simulink model "PubIfDecisionLM_MDL"  (R2020b)
settings: configuration reference "DspaceConfig" (kept outside this file)
PostLoadFcn:
  | if any(exist('dsrtsu_mdlpostloadfcn', 'file') ~= 0), dsrtsu_mdlpostloadfcn('Execute', bdroot); end
InitFcn:
  | , if any(exist('dsmpb_private', 'file') ~= 0), dsmpb_private('dsmpb_mdlclblib', 'Init', bdroot); end,
undefined symbols (not defined in the file or in its folder): OFM_OBJ_FUSIONTYPE_E, OFM_OBJ_MOVINGSTATE_E, OFM_OBJ_ORIENTATION_E, OFM_OBJ_TYPE_E, P_LM_Cyc, P_LM_EMLHistKapRcdBufSize, P_LM_EMLHistTrajBaseDis, P_LM_EMLHistTrajPNum, P_LM_EMLKapCorrMaxThre, P_LM_EMLMinKapThre, P_LM_EMLPathDisDiffThre, P_LM_EMLQuaFiltPar, P_LM_EMLTurnActKapThre, P_LM_EMLValidQuaThre, P_LM_FntPath1Disgap, P_LM_FntPath1MinDis, P_LM_FntPath1Timegap, P_LM_FntPath2Disgap, P_LM_FntPath2MinDis, P_LM_FntPath2Timegap, P_LM_FntPath3Disgap, P_LM_FntPath3MinDis, P_LM_FntPath3Timegap, P_LM_FusBLParFiltP, P_LM_FusEVDifC2Thre, P_LM_FusEVOPath1AllVSLDisThre, P_LM_FusEVOPath1AllVSLLostNumThre, P_LM_FusEVOPath1AllVSLQuaThre, P_LM_FusEVOPath1OTLFacNLC, P_LM_FusOTLQuaThre, P_LM_FusOTLSW, P_LM_FusParC0Index, P_LM_FusParC1Index, P_LM_FusParC2Index, P_LM_FusParC3Index, P_LM_FusVSLQuaThre, P_LM_FusVSLSW, P_LM_FusVSLValidSteerWheerAngThre, P_LM_FusVSLValidVxvThre, P_LM_LaneWidth, P_LM_OTLBufTPInfoEvaFactor, P_LM_OTLObjNum, P_LM_OTLObjSelectAgeThre, P_LM_OTLObjSelectDxAssessVx, P_LM_OTLObjSelectDxThre, P_LM_OTLObjSelectVxThre, P_LM_OTLObjSelectVyAssessDx, P_LM_OTLObjSelectVyThre, P_LM_OTLTrajPntBaseDis, P_LM_OTLTrajStdThre, P_LM_VSLAvailLineNum, P_LM_VSLBLSDiffThre, P_LM_VSLBLSDisRatio, P_LM_VSLFusBLParFiltP_C1, P_LM_VSLFusBLParFiltP_C2, P_LM_VSLFusBLParFiltP_C3, P_LM_VSLFusBLParFiltP_Quality, P_LM_VSLHistTrajBaseDis, P_LM_VSLHistTrajPNum, P_LM_VSLLCC0diff ... (+18)
libraries: simulink x145, LM_LIB x43
(part 22 of 24)

== matlab function PubIfDecisionLM_MDL/Subsystem2/LM_OTL/LM_OTL_MovObjTrajFit/LM_OTL_BufTPAssess/LM_OTL_BufTrajEva/Subsystem7/MATLAB Function1 ==
  data: Offset output; Flg output; LM_OTLBufValidInfo input; LM_OTLDxVect input; LM_OTLDyVect input; LM_OTLSPPos input; LM_OTLEPPos input; LM_FntPath1Dis input; LM_FntPath2Dis input; LM_FntPath3Dis input; TpValidNum output; SPValidPos output; P_LM_OTLTrajStdThre input
function [Offset,Flg,TpValidNum,SPValidPos] = fcn(LM_OTLBufValidInfo,LM_OTLDxVect,LM_OTLDyVect,LM_OTLSPPos,LM_OTLEPPos,LM_FntPath1Dis,LM_FntPath2Dis,LM_FntPath3Dis, P_LM_OTLTrajStdThre)


%%第一段前车道线取点
Offset=single(zeros(3,1));
Flg=uint8(zeros(3,1));
TpValidNum=uint8(zeros(3,1));
SPValidPos=uint8(zeros(3,1));
t_pnum=uint8(0);
t_sumy=single(0);
t_sumerry=single(0);
t_index=uint8(0);
if LM_OTLBufValidInfo(1)~=0
    if LM_OTLEPPos>=LM_OTLSPPos
        for i=LM_OTLSPPos:LM_OTLEPPos
            if LM_OTLDxVect(i)>0&&LM_OTLDxVect(i)<=LM_FntPath1Dis
                t_pnum=t_pnum+uint8(1);
                t_index=i;
                t_sumy=t_sumy+LM_OTLDyVect(i);
            end
        end
        t_mean=t_sumy/single(t_pnum);
        SPValidPos(1)=t_index-t_pnum+uint8(1);
        for i=t_index:-1:SPValidPos(1)
            t_error=(LM_OTLDyVect(i)-t_mean)^2;
            t_sumerry=t_sumerry+t_error;
        end
        if sqrt(t_sumerry/single(t_pnum))<=P_LM_OTLTrajStdThre
           Offset(1)=t_mean;
           Flg(1)=uint8(1);
           TpValidNum(1)=t_pnum;
        end
    elseif LM_OTLEPPos<LM_OTLSPPos
        for i=LM_OTLSPPos:80
            if LM_OTLDxVect(i)>0&&LM_OTLDxVect(i)<=LM_FntPath1Dis
                t_pnum=t_pnum+uint8(1);
                t_index=i;
                t_sumy=t_sumy+LM_OTLDyVect(i);
            end
        end
        for i=1:LM_OTLEPPos 
            if LM_OTLDxVect(i)>0&&LM_OTLDxVect(i)<=LM_FntPath1Dis
                t_pnum=t_pnum+uint8(1);
                t_index=i;
                t_sumy=t_sumy+LM_OTLDyVect(i);
            end
        end
        SPValidPos(1)=uint8(81)+t_index-t_pnum;
        t_mean=t_sumy/single(t_pnum);
        if SPValidPos(1)>80
            SPValidPos(1)=SPValidPos(1)-80;
        end
        if (SPValidPos(1)>=LM_OTLSPPos&&t_index>=LM_OTLSPPos)||(SPValidPos(1)<LM_OTLSPPos&&t_index<LM_OTLSPPos)
            for i=t_index:-1:SPValidPos(1)
                t_error=(LM_OTLDyVect(i)-t_mean)^2;
                t_sumerry=t_sumerry+t_error;
            end
        else
            for i=1:t_index
                t_error=(LM_OTLDyVect(i)-t_mean)^2;
                t_sumerry=t_sumerry+t_error;
            end
            for i=80:-1:SPValidPos(1)
                 t_error=(LM_OTLDyVect(i)-t_mean)^2;
                t_sumerry=t_sumerry+t_error;
            end
        end
        if sqrt(t_sumerry/single(t_pnum))<=P_LM_OTLTrajStdThre
           Offset(1)=t_mean;
           Flg(1)=uint8(1);
           TpValidNum(1)=t_pnum;
        end           
    end
end
%%第二段前车道线取点
t_pnum=uint8(0);
t_sumy=single(0);
t_sumerry=single(0);
t_index=uint8(0);
if LM_OTLBufValidInfo(2)~=0
    if LM_OTLEPPos>=LM_OTLSPPos
        for i=LM_OTLSPPos:LM_OTLEPPos
            if LM_OTLDxVect(i)>LM_FntPath1Dis&&LM_OTLDxVect(i)<=LM_FntPath2Dis
                t_pnum=t_pnum+uint8(1);
                t_index=i;
                t_sumy=t_sumy+LM_OTLDyVect(i);
            end
        end
        t_mean=t_sumy/single(t_pnum);
        SPValidPos(2)=t_index-t_pnum+uint8(1);
        for i=t_index:-1:SPValidPos(2)
            t_error=(LM_OTLDyVect(i)-t_mean)^2;
            t_sumerry=t_sumerry+t_error;
        end
        if sqrt(t_sumerry/single(t_pnum))<=P_LM_OTLTrajStdThre
           Offset(2)=t_mean;
           Flg(2)=uint8(1);
           TpValidNum(2)=t_pnum;
        end
    elseif LM_OTLEPPos<LM_OTLSPPos
        for i=LM_OTLSPPos:80
            if LM_OTLDxVect(i)>LM_FntPath1Dis&&LM_OTLDxVect(i)<=LM_FntPath2Dis
                t_pnum=t_pnum+uint8(1);
                t_index=i;
                t_sumy=t_sumy+LM_OTLDyVect(i);
            end
        end
        for i=1:LM_OTLEPPos 
            if LM_OTLDxVect(i)>LM_FntPath1Dis&&LM_OTLDxVect(i)<=LM_FntPath2Dis
                t_pnum=t_pnum+uint8(1);
                t_index=i;
                t_sumy=t_sumy+LM_OTLDyVect(i);
            end
        end
        t_mean=t_sumy/single(t_pnum);
        SPValidPos(2)=uint8(81)+t_index-t_pnum;
        if SPValidPos(2)>80
            SPValidPos(2)=SPValidPos(2)-80;
        end
        if (SPValidPos(2)>=LM_OTLSPPos&&t_index>=LM_OTLSPPos)||(SPValidPos(2)<LM_OTLSPPos&&t_index<LM_OTLSPPos)
            for i=t_index:-1:SPValidPos(2)
                t_error=(LM_OTLDyVect(i)-t_mean)^2;
                t_sumerry=t_sumerry+t_error;
            end
        else
            for i=1:t_index
                t_error=(LM_OTLDyVect(i)-t_mean)^2;
                t_sumerry=t_sumerry+t_error;
            end
            for i=80:-1:SPValidPos(2)
                t_error=(LM_OTLDyVect(i)-t_mean)^2;
                t_sumerry=t_sumerry+t_error;
            end
        end
        if sqrt(t_sumerry/single(t_pnum))<=P_LM_OTLTrajStdThre
           Offset(2)=t_mean;
           Flg(2)=uint8(1);
           TpValidNum(2)=t_pnum;
        end           
    end
end
%%第三段前车道线取点
t_pnum=uint8(0);
t_sumy=single(0);
t_sumerry=single(0);
t_index=uint8(0);
if LM_OTLBufValidInfo(3)~=0
    if LM_OTLEPPos>=LM_OTLSPPos
        for i=LM_OTLSPPos:LM_OTLEPPos
            if LM_OTLDxVect(i)>LM_FntPath2Dis&&LM_OTLDxVect(i)<=LM_FntPath3Dis
                t_pnum=t_pnum+uint8(1);
                t_index=i;
                t_sumy=t_sumy+LM_OTLDyVect(i);
            end
        end
        SPValidPos(3)=t_index-t_pnum+1;
        t_mean=t_sumy/single(t_pnum);
        for i=t_index:-1:SPValidPos(3)
            t_error=(LM_OTLDyVect(i)-t_mean)^2;
            t_sumerry=t_sumerry+t_error;
        end
        if sqrt(t_sumerry/single(t_pnum))<=P_LM_OTLTrajStdThre
           Offset(3)=t_mean;
           Flg(3)=uint8(1);
           TpValidNum(3)=t_pnum;
        end
    elseif LM_OTLEPPos<LM_OTLSPPos
        for i=LM_OTLSPPos:80
            if LM_OTLDxVect(i)>LM_FntPath2Dis&&LM_OTLDxVect(i)<=LM_FntPath3Dis
                t_pnum=t_pnum+uint8(1);
                t_index=i;
                t_sumy=t_sumy+LM_OTLDyVect(i);
            end
        end
        for i=1:LM_OTLEPPos 
            if LM_OTLDxVect(i)>LM_FntPath2Dis&&LM_OTLDxVect(i)<=LM_FntPath3Dis
                t_pnum=t_pnum+uint8(1);
                t_index=i;
                t_sumy=t_sumy+LM_OTLDyVect(i);
            end
        end
        t_mean=t_sumy/single(t_pnum);
        SPValidPos(3)=uint8(81)+t_index-t_pnum;
        if SPValidPos(3)>80
            SPValidPos(3)=SPValidPos(3)-80;
        end
        if (SPValidPos(3)>=LM_OTLSPPos&&t_index>=LM_OTLSPPos)||(SPValidPos(3)<LM_OTLSPPos&&t_index<LM_OTLSPPos)
            for i=t_index:-1:SPValidPos(3)
                t_error=(LM_OTLDyVect(i)-t_mean)^2;
                t_sumerry=t_sumerry+t_error;
            end
        else
            for i=1:t_index
                t_error=(LM_OTLDyVect(i)-t_mean)^2;
                t_sumerry=t_sumerry+t_error;
            end
            for i=80:-1:SPValidPos(3)
                t_error=(LM_OTLDyVect(i)-t_mean)^2;
                t_sumerry=t_sumerry+t_error;
            end
        end
        if sqrt(t_sumerry/single(t_pnum))<=P_LM_OTLTrajStdThre
           Offset(3)=t_mean;
           Flg(3)=uint8(1);
           TpValidNum(3)=t_pnum;
        end           
    end
end
end

== matlab function PubIfDecisionLM_MDL/Subsystem2/LM_OTL/LM_OTL_MovObjTrajFit/LM_OTL_BufTPAssess/LM_OTL_BufTrajEva/Subsystem8/MATLAB Function1 ==
  data: Offset output; Flg output; LM_OTLBufValidInfo input; LM_OTLDxVect input; LM_OTLDyVect input; LM_OTLSPPos input; LM_OTLEPPos input; LM_FntPath1Dis input; LM_FntPath2Dis input; LM_FntPath3Dis input; TpValidNum output; SPValidPos output; P_LM_OTLTrajStdThre input
function [Offset,Flg,TpValidNum,SPValidPos] = fcn(LM_OTLBufValidInfo,LM_OTLDxVect,LM_OTLDyVect,LM_OTLSPPos,LM_OTLEPPos,LM_FntPath1Dis,LM_FntPath2Dis,LM_FntPath3Dis, P_LM_OTLTrajStdThre)


%%第一段前车道线取点
Offset=single(zeros(3,1));
Flg=uint8(zeros(3,1));
TpValidNum=uint8(zeros(3,1));
SPValidPos=uint8(zeros(3,1));
t_pnum=uint8(0);
t_sumy=single(0);
t_sumerry=single(0);
t_index=uint8(0);
if LM_OTLBufValidInfo(1)~=0
    if LM_OTLEPPos>=LM_OTLSPPos
        for i=LM_OTLSPPos:LM_OTLEPPos
            if LM_OTLDxVect(i)>0&&LM_OTLDxVect(i)<=LM_FntPath1Dis
                t_pnum=t_pnum+uint8(1);
                t_index=i;
                t_sumy=t_sumy+LM_OTLDyVect(i);
            end
        end
        t_mean=t_sumy/single(t_pnum);
        SPValidPos(1)=t_index-t_pnum+uint8(1);
        for i=t_index:-1:SPValidPos(1)
            t_error=(LM_OTLDyVect(i)-t_mean)^2;
            t_sumerry=t_sumerry+t_error;
        end
        if sqrt(t_sumerry/single(t_pnum))<=P_LM_OTLTrajStdThre
           Offset(1)=t_mean;
           Flg(1)=uint8(1);
           TpValidNum(1)=t_pnum;
        end
    elseif LM_OTLEPPos<LM_OTLSPPos
        for i=LM_OTLSPPos:80
            if LM_OTLDxVect(i)>0&&LM_OTLDxVect(i)<=LM_FntPath1Dis
                t_pnum=t_pnum+uint8(1);
                t_index=i;
                t_sumy=t_sumy+LM_OTLDyVect(i);
            end
        end
        for i=1:LM_OTLEPPos 
            if LM_OTLDxVect(i)>0&&LM_OTLDxVect(i)<=LM_FntPath1Dis
                t_pnum=t_pnum+uint8(1);
                t_index=i;
                t_sumy=t_sumy+LM_OTLDyVect(i);
            end
        end
        SPValidPos(1)=uint8(81)+t_index-t_pnum;
        t_mean=t_sumy/single(t_pnum);
        if SPValidPos(1)>80
            SPValidPos(1)=SPValidPos(1)-80;
        end
        if (SPValidPos(1)>=LM_OTLSPPos&&t_index>=LM_OTLSPPos)||(SPValidPos(1)<LM_OTLSPPos&&t_index<LM_OTLSPPos)
            for i=t_index:-1:SPValidPos(1)
                t_error=(LM_OTLDyVect(i)-t_mean)^2;
                t_sumerry=t_sumerry+t_error;
            end
        else
            for i=1:t_index
                t_error=(LM_OTLDyVect(i)-t_mean)^2;
                t_sumerry=t_sumerry+t_error;
            end
            for i=80:-1:SPValidPos(1)
                 t_error=(LM_OTLDyVect(i)-t_mean)^2;
                t_sumerry=t_sumerry+t_error;
            end
        end
        if sqrt(t_sumerry/single(t_pnum))<=P_LM_OTLTrajStdThre
           Offset(1)=t_mean;
           Flg(1)=uint8(1);
           TpValidNum(1)=t_pnum;
        end           
    end
end
%%第二段前车道线取点
t_pnum=uint8(0);
t_sumy=single(0);
t_sumerry=single(0);
t_index=uint8(0);
if LM_OTLBufValidInfo(2)~=0
    if LM_OTLEPPos>=LM_OTLSPPos
        for i=LM_OTLSPPos:LM_OTLEPPos
            if LM_OTLDxVect(i)>LM_FntPath1Dis&&LM_OTLDxVect(i)<=LM_FntPath2Dis
                t_pnum=t_pnum+uint8(1);
                t_index=i;
                t_sumy=t_sumy+LM_OTLDyVect(i);
            end
        end
        t_mean=t_sumy/single(t_pnum);
        SPValidPos(2)=t_index-t_pnum+uint8(1);
        for i=t_index:-1:SPValidPos(2)
            t_error=(LM_OTLDyVect(i)-t_mean)^2;
            t_sumerry=t_sumerry+t_error;
        end
        if sqrt(t_sumerry/single(t_pnum))<=P_LM_OTLTrajStdThre
           Offset(2)=t_mean;
           Flg(2)=uint8(1);
           TpValidNum(2)=t_pnum;
        end
    elseif LM_OTLEPPos<LM_OTLSPPos
        for i=LM_OTLSPPos:80
            if LM_OTLDxVect(i)>LM_FntPath1Dis&&LM_OTLDxVect(i)<=LM_FntPath2Dis
                t_pnum=t_pnum+uint8(1);
                t_index=i;
                t_sumy=t_sumy+LM_OTLDyVect(i);
            end
        end
        for i=1:LM_OTLEPPos 
            if LM_OTLDxVect(i)>LM_FntPath1Dis&&LM_OTLDxVect(i)<=LM_FntPath2Dis
                t_pnum=t_pnum+uint8(1);
                t_index=i;
                t_sumy=t_sumy+LM_OTLDyVect(i);
            end
        end
        t_mean=t_sumy/single(t_pnum);
        SPValidPos(2)=uint8(81)+t_index-t_pnum;
        if SPValidPos(2)>80
            SPValidPos(2)=SPValidPos(2)-80;
        end
        if (SPValidPos(2)>=LM_OTLSPPos&&t_index>=LM_OTLSPPos)||(SPValidPos(2)<LM_OTLSPPos&&t_index<LM_OTLSPPos)
            for i=t_index:-1:SPValidPos(2)
                t_error=(LM_OTLDyVect(i)-t_mean)^2;
                t_sumerry=t_sumerry+t_error;
            end
        else
            for i=1:t_index
                t_error=(LM_OTLDyVect(i)-t_mean)^2;
                t_sumerry=t_sumerry+t_error;
            end
            for i=80:-1:SPValidPos(2)
                t_error=(LM_OTLDyVect(i)-t_mean)^2;
                t_sumerry=t_sumerry+t_error;
            end
        end
        if sqrt(t_sumerry/single(t_pnum))<=P_LM_OTLTrajStdThre
           Offset(2)=t_mean;
           Flg(2)=uint8(1);
           TpValidNum(2)=t_pnum;
        end           
    end
end
%%第三段前车道线取点
t_pnum=uint8(0);
t_sumy=single(0);
t_sumerry=single(0);
t_index=uint8(0);
if LM_OTLBufValidInfo(3)~=0
    if LM_OTLEPPos>=LM_OTLSPPos
        for i=LM_OTLSPPos:LM_OTLEPPos
            if LM_OTLDxVect(i)>LM_FntPath2Dis&&LM_OTLDxVect(i)<=LM_FntPath3Dis
                t_pnum=t_pnum+uint8(1);
                t_index=i;
                t_sumy=t_sumy+LM_OTLDyVect(i);
            end
        end
        SPValidPos(3)=t_index-t_pnum+1;
        t_mean=t_sumy/single(t_pnum);
        for i=t_index:-1:SPValidPos(3)
            t_error=(LM_OTLDyVect(i)-t_mean)^2;
            t_sumerry=t_sumerry+t_error;
        end
        if sqrt(t_sumerry/single(t_pnum))<=P_LM_OTLTrajStdThre
           Offset(3)=t_mean;
           Flg(3)=uint8(1);
           TpValidNum(3)=t_pnum;
        end
    elseif LM_OTLEPPos<LM_OTLSPPos
        for i=LM_OTLSPPos:80
            if LM_OTLDxVect(i)>LM_FntPath2Dis&&LM_OTLDxVect(i)<=LM_FntPath3Dis
                t_pnum=t_pnum+uint8(1);
                t_index=i;
                t_sumy=t_sumy+LM_OTLDyVect(i);
            end
        end
        for i=1:LM_OTLEPPos 
            if LM_OTLDxVect(i)>LM_FntPath2Dis&&LM_OTLDxVect(i)<=LM_FntPath3Dis
                t_pnum=t_pnum+uint8(1);
                t_index=i;
                t_sumy=t_sumy+LM_OTLDyVect(i);
            end
        end
        t_mean=t_sumy/single(t_pnum);
        SPValidPos(3)=uint8(81)+t_index-t_pnum;
        if SPValidPos(3)>80
            SPValidPos(3)=SPValidPos(3)-80;
        end
        if (SPValidPos(3)>=LM_OTLSPPos&&t_index>=LM_OTLSPPos)||(SPValidPos(3)<LM_OTLSPPos&&t_index<LM_OTLSPPos)
            for i=t_index:-1:SPValidPos(3)
                t_error=(LM_OTLDyVect(i)-t_mean)^2;
                t_sumerry=t_sumerry+t_error;
            end
        else
            for i=1:t_index
                t_error=(LM_OTLDyVect(i)-t_mean)^2;
                t_sumerry=t_sumerry+t_error;
            end
            for i=80:-1:SPValidPos(3)
                t_error=(LM_OTLDyVect(i)-t_mean)^2;
                t_sumerry=t_sumerry+t_error;
            end
        end
        if sqrt(t_sumerry/single(t_pnum))<=P_LM_OTLTrajStdThre
           Offset(3)=t_mean;
           Flg(3)=uint8(1);
           TpValidNum(3)=t_pnum;
        end           
    end
end
end

== matlab function PubIfDecisionLM_MDL/Subsystem2/LM_OTL/LM_OTL_MovObjTrajFit/LM_OTL_BufTPAssess/LM_OTL_BufTrajEva/Subsystem9/MATLAB Function1 ==
  data: Offset output; Flg output; LM_OTLBufValidInfo input; LM_OTLDxVect input; LM_OTLDyVect input; LM_OTLSPPos input; LM_OTLEPPos input; LM_FntPath1Dis input; LM_FntPath2Dis input; LM_FntPath3Dis input; TpValidNum output; SPValidPos output; P_LM_OTLTrajStdThre input
function [Offset,Flg,TpValidNum,SPValidPos] = fcn(LM_OTLBufValidInfo,LM_OTLDxVect,LM_OTLDyVect,LM_OTLSPPos,LM_OTLEPPos,LM_FntPath1Dis,LM_FntPath2Dis,LM_FntPath3Dis, P_LM_OTLTrajStdThre)


%%第一段前车道线取点
Offset=single(zeros(3,1));
Flg=uint8(zeros(3,1));
TpValidNum=uint8(zeros(3,1));
SPValidPos=uint8(zeros(3,1));
t_pnum=uint8(0);
t_sumy=single(0);
t_sumerry=single(0);
t_index=uint8(0);
if LM_OTLBufValidInfo(1)~=0
    if LM_OTLEPPos>=LM_OTLSPPos
        for i=LM_OTLSPPos:LM_OTLEPPos
            if LM_OTLDxVect(i)>0&&LM_OTLDxVect(i)<=LM_FntPath1Dis
                t_pnum=t_pnum+uint8(1);
                t_index=i;
                t_sumy=t_sumy+LM_OTLDyVect(i);
            end
        end
        t_mean=t_sumy/single(t_pnum);
        SPValidPos(1)=t_index-t_pnum+uint8(1);
        for i=t_index:-1:SPValidPos(1)
            t_error=(LM_OTLDyVect(i)-t_mean)^2;
            t_sumerry=t_sumerry+t_error;
        end
        if sqrt(t_sumerry/single(t_pnum))<=P_LM_OTLTrajStdThre
           Offset(1)=t_mean;
           Flg(1)=uint8(1);
           TpValidNum(1)=t_pnum;
        end
    elseif LM_OTLEPPos<LM_OTLSPPos
        for i=LM_OTLSPPos:80
            if LM_OTLDxVect(i)>0&&LM_OTLDxVect(i)<=LM_FntPath1Dis
                t_pnum=t_pnum+uint8(1);
                t_index=i;
                t_sumy=t_sumy+LM_OTLDyVect(i);
            end
        end
        for i=1:LM_OTLEPPos 
            if LM_OTLDxVect(i)>0&&LM_OTLDxVect(i)<=LM_FntPath1Dis
                t_pnum=t_pnum+uint8(1);
                t_index=i;
                t_sumy=t_sumy+LM_OTLDyVect(i);
            end
        end
        SPValidPos(1)=uint8(81)+t_index-t_pnum;
        t_mean=t_sumy/single(t_pnum);
        if SPValidPos(1)>80
            SPValidPos(1)=SPValidPos(1)-80;
        end
        if (SPValidPos(1)>=LM_OTLSPPos&&t_index>=LM_OTLSPPos)||(SPValidPos(1)<LM_OTLSPPos&&t_index<LM_OTLSPPos)
            for i=t_index:-1:SPValidPos(1)
                t_error=(LM_OTLDyVect(i)-t_mean)^2;
                t_sumerry=t_sumerry+t_error;
            end
        else
            for i=1:t_index
                t_error=(LM_OTLDyVect(i)-t_mean)^2;
                t_sumerry=t_sumerry+t_error;
            end
            for i=80:-1:SPValidPos(1)
                 t_error=(LM_OTLDyVect(i)-t_mean)^2;
                t_sumerry=t_sumerry+t_error;
            end
        end
        if sqrt(t_sumerry/single(t_pnum))<=P_LM_OTLTrajStdThre
           Offset(1)=t_mean;
           Flg(1)=uint8(1);
           TpValidNum(1)=t_pnum;
        end           
    end
end
%%第二段前车道线取点
t_pnum=uint8(0);
t_sumy=single(0);
t_sumerry=single(0);
t_index=uint8(0);
if LM_OTLBufValidInfo(2)~=0
    if LM_OTLEPPos>=LM_OTLSPPos
        for i=LM_OTLSPPos:LM_OTLEPPos
            if LM_OTLDxVect(i)>LM_FntPath1Dis&&LM_OTLDxVect(i)<=LM_FntPath2Dis
                t_pnum=t_pnum+uint8(1);
                t_index=i;
                t_sumy=t_sumy+LM_OTLDyVect(i);
            end
        end
        t_mean=t_sumy/single(t_pnum);
        SPValidPos(2)=t_index-t_pnum+uint8(1);
        for i=t_index:-1:SPValidPos(2)
            t_error=(LM_OTLDyVect(i)-t_mean)^2;
            t_sumerry=t_sumerry+t_error;
        end
        if sqrt(t_sumerry/single(t_pnum))<=P_LM_OTLTrajStdThre
           Offset(2)=t_mean;
           Flg(2)=uint8(1);
           TpValidNum(2)=t_pnum;
        end
    elseif LM_OTLEPPos<LM_OTLSPPos
        for i=LM_OTLSPPos:80
            if LM_OTLDxVect(i)>LM_FntPath1Dis&&LM_OTLDxVect(i)<=LM_FntPath2Dis
                t_pnum=t_pnum+uint8(1);
                t_index=i;
                t_sumy=t_sumy+LM_OTLDyVect(i);
            end
        end
        for i=1:LM_OTLEPPos 
            if LM_OTLDxVect(i)>LM_FntPath1Dis&&LM_OTLDxVect(i)<=LM_FntPath2Dis
                t_pnum=t_pnum+uint8(1);
                t_index=i;
                t_sumy=t_sumy+LM_OTLDyVect(i);
            end
        end
        t_mean=t_sumy/single(t_pnum);
        SPValidPos(2)=uint8(81)+t_index-t_pnum;
        if SPValidPos(2)>80
            SPValidPos(2)=SPValidPos(2)-80;
        end
        if (SPValidPos(2)>=LM_OTLSPPos&&t_index>=LM_OTLSPPos)||(SPValidPos(2)<LM_OTLSPPos&&t_index<LM_OTLSPPos)
            for i=t_index:-1:SPValidPos(2)
                t_error=(LM_OTLDyVect(i)-t_mean)^2;
                t_sumerry=t_sumerry+t_error;
            end
        else
            for i=1:t_index
                t_error=(LM_OTLDyVect(i)-t_mean)^2;
                t_sumerry=t_sumerry+t_error;
            end
            for i=80:-1:SPValidPos(2)
                t_error=(LM_OTLDyVect(i)-t_mean)^2;
                t_sumerry=t_sumerry+t_error;
            end
        end
        if sqrt(t_sumerry/single(t_pnum))<=P_LM_OTLTrajStdThre
           Offset(2)=t_mean;
           Flg(2)=uint8(1);
           TpValidNum(2)=t_pnum;
        end           
    end
end
%%第三段前车道线取点
t_pnum=uint8(0);
t_sumy=single(0);
t_sumerry=single(0);
t_index=uint8(0);
if LM_OTLBufValidInfo(3)~=0
    if LM_OTLEPPos>=LM_OTLSPPos
        for i=LM_OTLSPPos:LM_OTLEPPos
            if LM_OTLDxVect(i)>LM_FntPath2Dis&&LM_OTLDxVect(i)<=LM_FntPath3Dis
                t_pnum=t_pnum+uint8(1);
                t_index=i;
                t_sumy=t_sumy+LM_OTLDyVect(i);
            end
        end
        SPValidPos(3)=t_index-t_pnum+1;
        t_mean=t_sumy/single(t_pnum);
        for i=t_index:-1:SPValidPos(3)
            t_error=(LM_OTLDyVect(i)-t_mean)^2;
            t_sumerry=t_sumerry+t_error;
        end
        if sqrt(t_sumerry/single(t_pnum))<=P_LM_OTLTrajStdThre
           Offset(3)=t_mean;
           Flg(3)=uint8(1);
           TpValidNum(3)=t_pnum;
        end
    elseif LM_OTLEPPos<LM_OTLSPPos
        for i=LM_OTLSPPos:80
            if LM_OTLDxVect(i)>LM_FntPath2Dis&&LM_OTLDxVect(i)<=LM_FntPath3Dis
                t_pnum=t_pnum+uint8(1);
                t_index=i;
                t_sumy=t_sumy+LM_OTLDyVect(i);
            end
        end
        for i=1:LM_OTLEPPos 
            if LM_OTLDxVect(i)>LM_FntPath2Dis&&LM_OTLDxVect(i)<=LM_FntPath3Dis
                t_pnum=t_pnum+uint8(1);
                t_index=i;
                t_sumy=t_sumy+LM_OTLDyVect(i);
            end
        end
        t_mean=t_sumy/single(t_pnum);
        SPValidPos(3)=uint8(81)+t_index-t_pnum;
        if SPValidPos(3)>80
            SPValidPos(3)=SPValidPos(3)-80;
        end
        if (SPValidPos(3)>=LM_OTLSPPos&&t_index>=LM_OTLSPPos)||(SPValidPos(3)<LM_OTLSPPos&&t_index<LM_OTLSPPos)
            for i=t_index:-1:SPValidPos(3)
                t_error=(LM_OTLDyVect(i)-t_mean)^2;
                t_sumerry=t_sumerry+t_error;
            end
        else
            for i=1:t_index
                t_error=(LM_OTLDyVect(i)-t_mean)^2;
                t_sumerry=t_sumerry+t_error;
            end
            for i=80:-1:SPValidPos(3)
                t_error=(LM_OTLDyVect(i)-t_mean)^2;
                t_sumerry=t_sumerry+t_error;
            end
        end
        if sqrt(t_sumerry/single(t_pnum))<=P_LM_OTLTrajStdThre
           Offset(3)=t_mean;
           Flg(3)=uint8(1);
           TpValidNum(3)=t_pnum;
        end           
    end
end
end

== matlab function PubIfDecisionLM_MDL/Subsystem2/LM_OTL/LM_OTL_MovObjTrajFit/LM_OTL_TrajFit/MATLAB Function1 ==
  data: LM_OTLFntPath1P output; LM_OTLFntPath1Qulity output; LM_OTLFntPath2P output; LM_OTLFntPath2Qulity output; LM_OTLFntPath3P output; LM_OTLFntPath3Qulity output; LM_OTLBufResampeFntPathDxInfo input; LM_OTLBufResampeFntPathDyInfo input; LM_FntPath1Dis input; LM_FntPath2Dis input; LM_FntPath3Dis input
function [ LM_OTLFntPath1P,LM_OTLFntPath1Qulity,LM_OTLFntPath2P,LM_OTLFntPath2Qulity,LM_OTLFntPath3P,LM_OTLFntPath3Qulity] = ...
          fcn(LM_OTLBufResampeFntPathDxInfo,LM_OTLBufResampeFntPathDyInfo,LM_FntPath1Dis,LM_FntPath2Dis,LM_FntPath3Dis)

%%参数初始化     
P_LM_OTLHPFntBuffSize = uint8(80);
t_tpx = single(zeros(P_LM_OTLHPFntBuffSize,1));
t_tpy = single(zeros(P_LM_OTLHPFntBuffSize,1));
t_tpnum = uint8(1);
t_tp1num = uint8(0);
t_tp2num = uint8(0);
t_tp3num = uint8(0);
t_index1min=uint8(81);
t_index1max=uint8(0);
t_index2min=uint8(81);
t_index2max=uint8(0);
t_index3min=uint8(81);
t_index3max=uint8(0);
t_std=single(0);
%%车道线拟合
for i = 1:80
    if LM_OTLBufResampeFntPathDxInfo(i) < LM_FntPath3Dis && LM_OTLBufResampeFntPathDxInfo(i) >= 0
        if LM_OTLBufResampeFntPathDxInfo(i) ~= 0 && LM_OTLBufResampeFntPathDyInfo(i) ~= 0
            t_tpnum = t_tpnum + uint8(1);
            t_tpx(t_tpnum) = LM_OTLBufResampeFntPathDxInfo(i);
            t_tpy(t_tpnum) = LM_OTLBufResampeFntPathDyInfo(i);
        end
    end
end
if t_tpnum >= 8  %多于8个点进行拟合，否则不进行
    if t_tpnum < P_LM_OTLHPFntBuffSize
        for i = t_tpnum+1:P_LM_OTLHPFntBuffSize
            t_tpx(i) = t_tpx(t_tpnum);
            t_tpy(i) = t_tpy(t_tpnum);
        end
    end
    %车道线拟合
    LM_OTLFntPathP = polyfit(t_tpx,t_tpy,3);
    % 误差计算
    t_fity = polyval(LM_OTLFntPathP,t_tpx);
    t_sumerry = single(0);
    for i=1:t_tpnum
        t_erry = single((t_tpy(i) - t_fity(i))^2);
        t_sumerry = t_sumerry + t_erry;
    end
    t_std=sqrt(t_sumerry/single(t_tpnum));
    t_quality = interpolate(single(0.1),single(1),single(0.4),single(0),single(t_std));
    %由轨迹点个数求轨迹质量影响因子，当轨迹点小于8个时，轨迹质量影响因子为0；当轨迹点大于18个时，轨迹质量影响因子为1
    t_factor = interpolate(single(8),single(0),single(17),single(1),single(t_tpnum));
    %轨迹质量= 轨迹质量*轨迹质量影响因子
    LM_OTLFntPathQulity = single(t_quality * t_factor);
    LM_OTLFntPathQulity = min(LM_OTLFntPathQulity,0.95);
    
% 轨迹质量计算 考虑历史轨迹点长度，及拟合误差
%  LM_EMLRearPath1Qulity = single(0.9);
else 
    LM_OTLFntPathP = single([0 0 0 0]);
    LM_OTLFntPathQulity = single(0);  
end
%% 判断各个路段轨迹点的个数及最大最小值标志位
for i = 1:80
    if LM_OTLBufResampeFntPathDxInfo(i) < LM_FntPath1Dis && LM_OTLBufResampeFntPathDxInfo(i) >= 0
        if LM_OTLBufResampeFntPathDxInfo(i) ~= 0 && LM_OTLBufResampeFntPathDyInfo(i) ~= 0
            t_tp1num = t_tp1num + uint8(1);
            if i>t_index1max
                t_index1max=uint8(i);
            end
            if i<t_index1min
                t_index1min=uint8(i);
            end  
        end
    end
    if LM_OTLBufResampeFntPathDxInfo(i) < LM_FntPath2Dis && LM_OTLBufResampeFntPathDxInfo(i) >= LM_FntPath1Dis
        if LM_OTLBufResampeFntPathDxInfo(i) ~= 0 && LM_OTLBufResampeFntPathDyInfo(i) ~= 0
            t_tp2num = t_tp2num + uint8(1);
            if i>t_index2max
                t_index2max=uint8(i);
            end
            if i<t_index2min
                t_index2min=uint8(i);
            end  
        end 
    end
    if LM_OTLBufResampeFntPathDxInfo(i) < LM_FntPath3Dis && LM_OTLBufResampeFntPathDxInfo(i) >= LM_FntPath2Dis
        if LM_OTLBufResampeFntPathDxInfo(i) ~= 0 && LM_OTLBufResampeFntPathDyInfo(i) ~= 0
            t_tp3num = t_tp3num + uint8(1);
            if i>t_index3max
                t_index3max=uint8(i);
            end
            if i<t_index3min
                t_index3min=uint8(i);
            end 
        end  
    end
end
%%质量计算
if t_tp1num~=0
    if t_tp2num~=0||t_tp3num~=0
        t_ratio=(LM_FntPath1Dis-LM_OTLBufResampeFntPathDxInfo(t_index1min))/LM_FntPath1Dis;
        t_factor = interpolate(single(0),single(0),single(1),single(1),single(t_ratio));
        LM_OTLFntPath1P = LM_OTLFntPathP ;
        LM_OTLFntPath1Qulity =t_factor*LM_OTLFntPathQulity;
    else
         t_ratio=(LM_OTLBufResampeFntPathDxInfo(t_index1max)-LM_OTLBufResampeFntPathDxInfo(t_index1min))/LM_FntPath1Dis;
         t_factor = interpolate(single(0),single(0),single(1),single(1),single(t_ratio));
         LM_OTLFntPath1P = LM_OTLFntPathP ;
         LM_OTLFntPath1Qulity =t_factor*LM_OTLFntPathQulity;
    end
    t_C0 = abs(LM_OTLFntPath1P(4));
    t_factor = interpolate(single(1),single(1),single(3),single(0),single(t_C0));
    LM_OTLFntPath1Qulity=t_factor*LM_OTLFntPath1Qulity;
else
    LM_OTLFntPath1P = single([0 0 0 0]);
    LM_OTLFntPath1Qulity = single(0);  
end
if t_tp3num~=0
    if t_tp1num~=0||t_tp2num~=0
        t_ratio=(LM_OTLBufResampeFntPathDxInfo(t_index3max)-LM_FntPath2Dis)/(LM_FntPath3Dis-LM_FntPath2Dis);
        t_factor = interpolate(single(0),single(0),single(1),single(1),single(t_ratio));
        LM_OTLFntPath3P = LM_OTLFntPathP ;
        LM_OTLFntPath3Qulity =t_factor*LM_OTLFntPathQulity;
    else
         t_ratio=(LM_OTLBufResampeFntPathDxInfo(t_index3max)-LM_OTLBufResampeFntPathDxInfo(t_index3min))/(LM_FntPath3Dis-LM_FntPath2Dis);
         t_factor = interpolate(single(0),single(0),single(1),single(1),single(t_ratio));
         LM_OTLFntPath3P = LM_OTLFntPathP ;
         LM_OTLFntPath3Qulity =t_factor*LM_OTLFntPathQulity;
    end
else
    LM_OTLFntPath3P = single([0 0 0 0]);
    LM_OTLFntPath3Qulity = single(0);  
end
if t_tp1num~=0&&t_tp3num~=0
    LM_OTLFntPath2P = LM_OTLFntPathP ;
    LM_OTLFntPath2Qulity = LM_OTLFntPathQulity;
elseif t_tp1num==0&&t_tp3num==0&&t_tp2num~=0
    t_ratio=(LM_OTLBufResampeFntPathDxInfo(t_index2max)-LM_OTLBufResampeFntPathDxInfo(t_index2min))/(LM_FntPath2Dis-LM_FntPath1Dis);
    t_factor = interpolate(single(0),single(0),single(1),single(1),single(t_ratio));
    LM_OTLFntPath2P = LM_OTLFntPathP ;
    LM_OTLFntPath2Qulity =t_factor*LM_OTLFntPathQulity;
elseif t_tp1num~=0&&t_tp3num==0&&t_tp2num~=0
    t_ratio=(LM_OTLBufResampeFntPathDxInfo(t_index2max)-LM_FntPath1Dis)/(LM_FntPath2Dis-LM_FntPath1Dis);
    t_factor = interpolate(single(0),single(0),single(1),single(1),single(t_ratio));
    LM_OTLFntPath2P = LM_OTLFntPathP ;
    LM_OTLFntPath2Qulity =t_factor*LM_OTLFntPathQulity;
elseif t_tp1num==0&&t_tp3num~=0&&t_tp2num~=0
    t_ratio=(LM_FntPath2Dis-LM_OTLBufResampeFntPathDxInfo(t_index2min))/(LM_FntPath2Dis-LM_FntPath1Dis);
    t_factor = interpolate(single(0),single(0),single(1),single(1),single(t_ratio));
    LM_OTLFntPath2P = LM_OTLFntPathP ;
    LM_OTLFntPath2Qulity =t_factor*LM_OTLFntPathQulity;
else
    LM_OTLFntPath2P = single([0 0 0 0]);
    LM_OTLFntPath2Qulity = single(0);  
end

end
function out = interpolate(x1,z1,x2,z2,Raw)
if Raw<=x1
    out = single(z1);
else
    if Raw>=x2
        out = single(z2);
    else
        t_out = single((Raw-x1)*(z2-z1));
        t_out = single(t_out/(x2-x1));
        t_out = single(z1)+t_out;
        out = t_out;
    end
end
end
